simulink model "beta_estimator_velocity"  (R2017a)
settings: Solver=VariableStepAuto  StartTime=0.0  StopTime=10.0  RelTol=1e-3
undefined symbols (not defined in the file or in its folder): KD, KP, N
libraries: robotlib x4, simulink x2
settings Model: Creator=bascetta  LastModifiedBy=bascetta

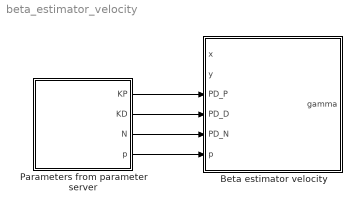
== system beta_estimator_velocity ==
  Beta estimator velocity : Subsystem
  Parameters from parameter server : Subsystem
  wires:
  Parameters from parameter server/1(KP) -> Beta estimator velocity/3(PD_P)
  Parameters from parameter server/2(KD) -> Beta estimator velocity/4(PD_D)
  Parameters from parameter server/3(N) -> Beta estimator velocity/5(PD_N)
  Parameters from parameter server/4(p) -> Beta estimator velocity/6(p)

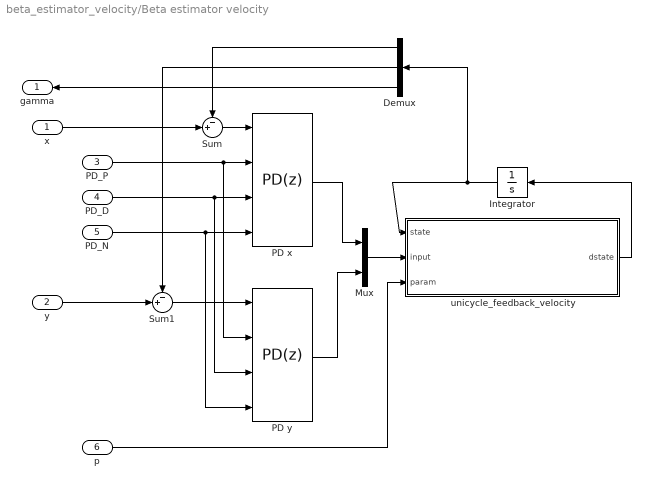
== system beta_estimator_velocity/Beta estimator velocity ==
  x : Inport
  y : Inport  Port=2
  PD_P : Inport  Port=3
  PD_D : Inport  Port=4
  PD_N : Inport  Port=5
  p : Inport  Port=6
  Demux : Demux  Outputs=3
  Integrator : Integrator
  Mux : Mux  Inputs=2
  PD x : simulink/Continuous/PID Controller  Controller=PD  TimeDomain=Discrete-time  SampleTime=-1  IntegratorMethod=Forward Euler  FilterMethod=Trapezoidal  Form=Parallel  UseFilter=on  ControllerParametersSource=external  P=KP  I=0  D=KD  N=N  InitialConditionSource=internal  InitialConditionForIntegrator=0  InitialConditionForFilter=0  ExternalReset=none  LimitOutput=off  UpperSaturationLimit=inf  LowerSaturationLimit=-inf  LinearizeAsGain=on  AntiWindupMode=none  Kb=1  TrackingMode=off  Kt=1  PParamMin=[]  PParamMax=[]  IParamMin=[]  IParamMax=[]  DParamMin=[]  DParamMax=[]  NParamMin=[]  NParamMax=[]  KbParamMin=[]  KbParamMax=[]  KtParamMin=[]  KtParamMax=[]  POutMin=[]  POutMax=[]  IOutMin=[]  IOutMax=[]  DOutMin=[]  DOutMax=[]  NOutMin=[]  NOutMax=[]  KbOutMin=[]  KbOutMax=[]  KtOutMin=[]  KtOutMax=[]  IntegratorOutMin=[]  IntegratorOutMax=[]  FilterOutMin=[]  FilterOutMax=[]  SumOutMin=[]  SumOutMax=[]  SumI1OutMin=[]  SumI1OutMax=[]  SumI2OutMin=[]  SumI2OutMax=[]  SumI3OutMin=[]  SumI3OutMax=[]  SumDOutMin=[]  SumDOutMax=[]  SaturationOutMin=[]  SaturationOutMax=[]  IntegratorContinuousStateAttributes=''  IntegratorStateMustResolveToSignalObject=off  IntegratorRTWStateStorageClass=Auto  FilterContinuousStateAttributes=''  FilterStateMustResolveToSignalObject=off  FilterRTWStateStorageClass=Auto  DifferentiatorICPrevScaledInput=0  DifferentiatorOutMin=[]  DifferentiatorOutMax=[]  InitialConditionSetting=State (most efficient)
  PD y : simulink/Continuous/PID Controller  Controller=PD  TimeDomain=Discrete-time  SampleTime=-1  IntegratorMethod=Forward Euler  FilterMethod=Trapezoidal  Form=Parallel  UseFilter=on  ControllerParametersSource=external  P=KP  I=0  D=KD  N=N  InitialConditionSource=internal  InitialConditionForIntegrator=0  InitialConditionForFilter=0  ExternalReset=none  LimitOutput=off  UpperSaturationLimit=inf  LowerSaturationLimit=-inf  LinearizeAsGain=on  AntiWindupMode=none  Kb=1  TrackingMode=off  Kt=1  PParamMin=[]  PParamMax=[]  IParamMin=[]  IParamMax=[]  DParamMin=[]  DParamMax=[]  NParamMin=[]  NParamMax=[]  KbParamMin=[]  KbParamMax=[]  KtParamMin=[]  KtParamMax=[]  POutMin=[]  POutMax=[]  IOutMin=[]  IOutMax=[]  DOutMin=[]  DOutMax=[]  NOutMin=[]  NOutMax=[]  KbOutMin=[]  KbOutMax=[]  KtOutMin=[]  KtOutMax=[]  IntegratorOutMin=[]  IntegratorOutMax=[]  FilterOutMin=[]  FilterOutMax=[]  SumOutMin=[]  SumOutMax=[]  SumI1OutMin=[]  SumI1OutMax=[]  SumI2OutMin=[]  SumI2OutMax=[]  SumI3OutMin=[]  SumI3OutMax=[]  SumDOutMin=[]  SumDOutMax=[]  SaturationOutMin=[]  SaturationOutMax=[]  IntegratorContinuousStateAttributes=''  IntegratorStateMustResolveToSignalObject=off  IntegratorRTWStateStorageClass=Auto  FilterContinuousStateAttributes=''  FilterStateMustResolveToSignalObject=off  FilterRTWStateStorageClass=Auto  DifferentiatorICPrevScaledInput=0  DifferentiatorOutMin=[]  DifferentiatorOutMax=[]  InitialConditionSetting=State (most efficient)
  Sum : Sum  Inputs=-+|
  Sum1 : Sum  Inputs=-+|
  unicycle_feedback_velocity : MATLAB Function  TreatAsAtomicUnit=on
  gamma : Outport
  wires:
  Demux/3 -> gamma/1
  PD_D/1 -> PD x/3, PD y/3
  y/1 -> Sum1/2
  PD_P/1 -> PD x/2, PD y/2
  Demux/1 -> Sum/1
  Sum1/1 -> PD y/1
  PD y/1 -> Mux/2
  PD x/1 -> Mux/1
  Mux/1 -> unicycle_feedback_velocity/2(input)
  p/1 -> unicycle_feedback_velocity/3(param)
  unicycle_feedback_velocity/1(dstate) -> Integrator/1
  Integrator/1 -> unicycle_feedback_velocity/1(state), Demux/1
  PD_N/1 -> PD x/4, PD y/4
  Sum/1 -> PD x/1
  Demux/2 -> Sum1/1
  x/1 -> Sum/2

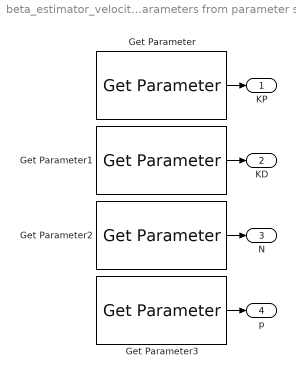
== system beta_estimator_velocity/Parameters from parameter server ==
  Get Parameter : robotlib/Get Parameter  SourceLibraryInfo=This block requires Robotics System Toolbox  ParameterSource=Specify your own  ParameterName=/beta_estimator/KP  ParameterType=double  ParameterMaxArrayLength=16  ParameterInitialValue=0.0  SampleTime=-1  ShowErrorCodeOutput=off  ModelName=beta_estimator_acceleration  BlockId=ParamGet_beta_estimator_acceleration_22
      settings: SourceProductName=Robotics System Toolbox  SourceProductBaseCode=RO
  Get Parameter1 : robotlib/Get Parameter  SourceLibraryInfo=This block requires Robotics System Toolbox  ParameterSource=Specify your own  ParameterName=/beta_estimator/KD  ParameterType=double  ParameterMaxArrayLength=16  ParameterInitialValue=0.0  SampleTime=-1  ShowErrorCodeOutput=off  ModelName=beta_estimator_acceleration  BlockId=ParamGet_beta_estimator_acceleration_23
      settings: SourceProductName=Robotics System Toolbox  SourceProductBaseCode=RO
  Get Parameter2 : robotlib/Get Parameter  SourceLibraryInfo=This block requires Robotics System Toolbox  ParameterSource=Specify your own  ParameterName=/beta_estimator/N  ParameterType=double  ParameterMaxArrayLength=16  ParameterInitialValue=0.0  SampleTime=-1  ShowErrorCodeOutput=off  ModelName=beta_estimator_acceleration  BlockId=ParamGet_beta_estimator_acceleration_24
      settings: SourceProductName=Robotics System Toolbox  SourceProductBaseCode=RO
  Get Parameter3 : robotlib/Get Parameter  SourceLibraryInfo=This block requires Robotics System Toolbox  ParameterSource=Specify your own  ParameterName=/beta_estimator/p  ParameterType=double  ParameterMaxArrayLength=16  ParameterInitialValue=0.0  SampleTime=-1  ShowErrorCodeOutput=off  ModelName=beta_estimator_velocity  BlockId=ParamGet_beta_estimator_velocity_63
      settings: SourceProductName=Robotics System Toolbox  SourceProductBaseCode=RO
  KP : Outport
  KD : Outport  Port=2
  N : Outport  Port=3
  p : Outport  Port=4
  wires:
  Get Parameter/1 -> KP/1
  Get Parameter2/1 -> N/1
  Get Parameter1/1 -> KD/1
  Get Parameter3/1 -> p/1

== matlab function beta_estimator_velocity/Beta estimator velocity/unicycle_feedback_velocity ==
  data: state input; dstate output; input input; param input
function dstate = unicycle_feedback_velocity(state,input,param)

% State and input variables
x     = state(1);
y     = state(1);
gamma = state(3); % theta+beta
vxp   = input(1);
vyp   = input(2);

% Parameters
p = param(1);

% Model equations
dstate = zeros(3,1);
dstate(1) = vxp*cos(gamma)^2+vyp*sin(gamma)*cos(gamma);
dstate(2) = vxp*sin(gamma)*cos(gamma)+vyp*sin(gamma)^2;
dstate(3) = (vyp*cos(gamma)-vxp*sin(gamma))/p;
